simulink model "DZ_DSMC"  (R2021b)
settings: Solver=FixedStepAuto  StartTime=0.0  StopTime=30  FixedStep=1e-5  MaxStep=0.015  RelTol=1e-3
PreLoadFcn:
  | if ~exist('sim_HIL')
  |     sim_HIL=false;
  | end
  | if ~exist('usefilter')
  |     usefilter=false;
  | end
InitFcn:
  | load motorModel.mat
  | load expsetup
model workspace (MAT data in the model file):
  C = Simulink.Parameter
  C.Value = Simulink.data.Expression
  C.Value.ExpressionString = "single(Cs(nodeID,:))"
  C.DataType = 'single'
  C.Complexity = 'real'
  C.Dimensions = -1
  Gam = Simulink.Parameter
  Gam.Value = Simulink.data.Expression
  Gam.Value.ExpressionString = "single(mModel{nodeID,3}.B)"
  Gam.DataType = 'single'
  Gam.Complexity = 'real'
  Gam.Dimensions = -1
  Phi = Simulink.Parameter
  Phi.Value = Simulink.data.Expression
  Phi.Value.ExpressionString = "single(mModel{nodeID,3}.A)"
  Phi.DataType = 'single'
  Phi.Complexity = 'real'
  Phi.Dimensions = -1
  del = Simulink.Parameter
  del.Value = Simulink.data.Expression
  del.Value.ExpressionString = "single(dels(nodeID))"
  del.DataType = 'single'
  del.Complexity = 'real'
  del.Dimensions = -1
  eta = Simulink.Parameter
  eta.Value = Simulink.data.Expression
  eta.Value.ExpressionString = "single(etas(nodeID))"
  eta.DataType = 'single'
  eta.Complexity = 'real'
  eta.Dimensions = -1
  gamm = Simulink.Parameter
  gamm.Value = Simulink.data.Expression
  gamm.Value.ExpressionString = "round(gamms(nodeID))"
  gamm.DataType = 'single'
  gamm.Complexity = 'real'
  gamm.Dimensions = -1
  qT = Simulink.Parameter
  qT.Value = Simulink.data.Expression
  qT.Value.ExpressionString = "single(qTs(nodeID))"
  qT.DataType = 'single'
  qT.Complexity = 'real'
  qT.Dimensions = -1
  vphi = Simulink.Parameter
  vphi.Value = Simulink.data.Expression
  vphi.Value.ExpressionString = "single(vphis(nodeID))"
  vphi.DataType = 'single'
  vphi.Complexity = 'real'
  vphi.Dimensions = -1
  xiT = Simulink.Parameter
  xiT.Value = Simulink.data.Expression
  xiT.Value.ExpressionString = "single(xiTs(nodeID))"
  xiT.DataType = 'single'
  xiT.Complexity = 'real'
  xiT.Dimensions = -1
undefined symbols (not defined in the file): DiscIntNeverNeededParam, N, nodeID, ss_sys, Ts, x607325_PPR
libraries: simulink x1
settings Model: DataDictionary=MotorInfo.sldd  SimulationMode=accelerator  CodeVerificationMode=processor-in-the-loop (pil)  ExtModeTrigDuration=2  Creator=khoi  LastModifiedBy=khoi
settings SolverCC: AlgebraicLoopSolver=TrustRegion  AutoInsertRateTranBlk=on
settings DataIOCC: ExternalInput=i1, i2  LoadExternalInput=on  SaveOutput=off  SaveTime=off
settings OptimizationCC: UseDivisionForNetSlopeComputation=on  GainParamInheritBuiltInType=on  UseFloatMulNetSlope=on  DefaultUnderspecifiedDataType=single  UseSpecifiedMinMax=on  StrengthReduction=on  BitwiseOrLogicalOp=Bitwise operator  PassReuseOutputArgsAs=Individual arguments  NoFixptDivByZeroProtection=on  EfficientFloat2IntCast=on  LifeSpan=inf  MaxStackSize=1024  OptimizeBlockOrder=speed  DifferentSizesBufferReuse=on  OptimizationPriority=Speed  MultiThreadedLoops=on  EfficientTunableParamExpr=on
settings DebuggingCC: SignalInfNanChecking=error  AlgebraicLoopMsg=none  IntegerOverflowMsg=error  ParameterTunabilityLossMsg=error  AssertControl=DisableAll  SFUndirectedBroadcastEventsDiag=error  SFMachineParentedDataDiag=warning
settings HardwareCC: ProdLongLongMode=on
settings ModelReferenceCC: EnableParallelModelReferenceBuilds=on  PropagateVarSize=During execution
settings SFSimCC: CompileTimeRecursionLimit=0  EnableRuntimeRecursion=off  MATLABDynamicMemAlloc=off
settings RTWCC: Description=Embedded Coder  SystemTargetFile=ert.tlc  TemplateMakefile=ert_default_tmf  Toolchain=MinGW64 | gmake (64-bit Windows)  BuildConfiguration=Faster Runs
settings CodeAppCC: ForceParamTrailComments=on  IgnoreCustomStorageClasses=off  OperatorAnnotations=on  SimulinkDataObjDesc=on  SFDataObjDesc=on  MATLABFcnDesc=on  InsertBlockDesc=on
settings ERTTargetCC: TargetLangStandard=C99 (ISO)  CodeReplacementLibrary=GNU C99 extensions  UtilityFuncGeneration=Shared location  CombineSignalStateStructs=on  CodeInterfacePackaging=Reusable function  SupportNonFinite=off  SupportComplex=off  ParenthesesLevel=Maximum  CastingMode=Standards  GenerateAllocFcn=on  GenerateSharedConstants=off  ExtModeTransport=3  ExtModeStaticAlloc=on  ExtModeStaticAllocSize=2048  ExtModeMexFile=ext_xcp  ExtModeIntrfLevel=Level2 - Open  RootIOFormat=Part of model data structure  ERTCustomFileTemplate=example_file_process.tlc

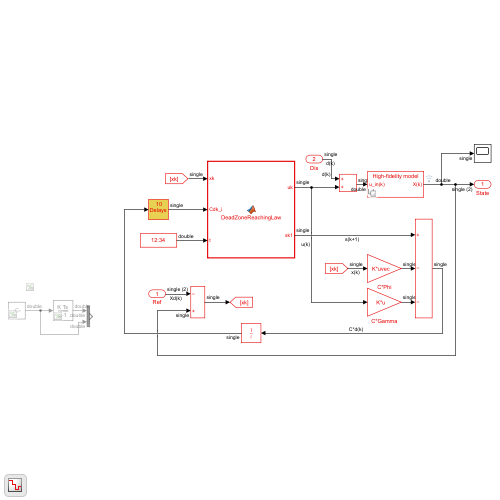
[thumbnail: Simulink's stored preview of the top-level diagram]
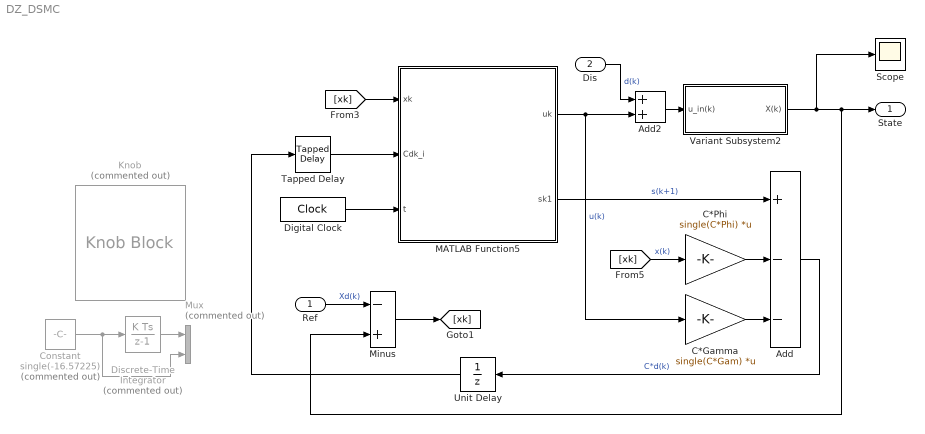
== system DZ_DSMC ==
  Ref : Inport  OutDataTypeStr=single  PortDimensions=2
  Dis : Inport  Port=2  OutDataTypeStr=single  PortDimensions=1
  Add : Sum  Inputs=+--
  Add2 : Sum  OutDataTypeStr=single
  C*Gamma : Gain  Gain=single(C*Gam)  Multiplication=Matrix(K*u)
  C*Phi : Gain  Gain=single(C*Phi)  Multiplication=Matrix(K*u) (u vector)
  Constant : Constant  Commented=on  Value=single(-16.57225)  SampleTime=Ts
  Digital Clock : DigitalClock  SampleTime=Ts
  Discrete-Time Integrator : DiscreteIntegrator  Commented=on  SampleTime=-1  ICPrevOutput=DiscIntNeverNeededParam  ICPrevScaledInput=DiscIntNeverNeededParam
  Knob : KnobBlock  Commented=on  ScaleMin=-50  ScaleMax=50
  MATLAB Function5 : MATLAB Function  TreatAsAtomicUnit=on  mask{Phi=single(Phi), Gam=single(Gam), C=single(C), qT=single(qT), xiT=single(xiT), del=single(del), vphi=single(vphi), gamm=uint8(gamm), eta=single(eta), Ts=single(Ts), n=uint8(N)}
      mask prompts: Gam "Gamma"; C "Sliding vector"; qT "qT (0<1-qT<1)"; xiT "xiT>0"; del "0<delta<1"; vphi "vphi>0"; gamm "gamma (natural num +)"; eta "eta>0"
  Minus : Sum  Inputs=-+
  Mux : Mux  Commented=on  Inputs=2
  Scope : Scope
  Tapped Delay : simulink/Discrete/Tapped Delay  vinit=0.0  samptime=-1  NumDelays=N  DelayOrder=Newest  includeCurrent=on
  Unit Delay : UnitDelay  SampleTime=-1  HasFrameUpgradeWarning=on
  Variant Subsystem2 : Subsystem  Variant=on  mask{Phi=single(Phi), Gam=single(Gam), NodeID=nodeID, Ts=single(Ts)}
      mask prompts: Phi "State matrix"; Gam "Input matrix"; NodeID "node ID"; Ts "Sample time (s)"
      mask init:
      | myDictionaryObj = Simulink.data.dictionary.open('MotorInfo.sldd');
      mask DialogControl ParameterGroupVar Prompt: Mathematical model
      mask DialogControl ParameterGroupVar_copy Prompt: Mathematical model
  State : Outport  OutDataTypeStr=single  PortDimensions=2
  wires:
  Minus/1 -> [xk]
  Add/1 -> Unit Delay/1  "C*d(k)"
  MATLAB Function5/1(uk) -> C*Gamma/1, Add2/2  "u(k)"
  [xk] -> MATLAB Function5/1(xk)
  [xk] -> C*Phi/1  "x(k)"
  MATLAB Function5/2(sk1) -> Add/1  "s(k+1)"
  C*Gamma/1 -> Add/3
  C*Phi/1 -> Add/2
  Tapped Delay/1 -> MATLAB Function5/2(Cdk_i)
  Dis/1 -> Add2/1  "d(k)"
  Unit Delay/1 -> Tapped Delay/1
  Digital Clock/1 -> MATLAB Function5/3(t)
  Ref/1 -> Minus/1  "Xd(k)"
  Discrete-Time Integrator/1 -> Mux/1
  Constant/1 -> Mux/2, Discrete-Time Integrator/1
  Variant Subsystem2/1(X(k)) -> Scope/1, Minus/2, State/1
  Add2/1 -> Variant Subsystem2/1(u_in(k))

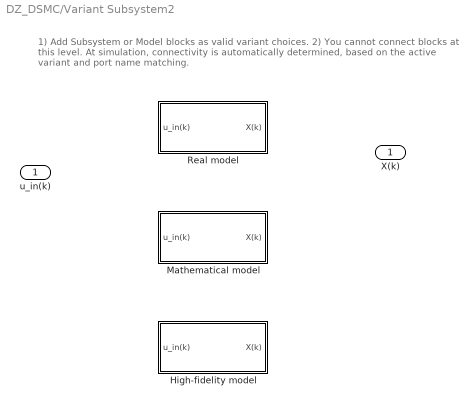
== system DZ_DSMC/Variant Subsystem2 ==
  note: 1) Add Subsystem or Model blocks as valid variant choices.
      | 2) You cannot connect blocks at this level. At simulation, connectivity is automatically
      | determined, based on the active variant and port name matching.
  u_in(k) : Inport
  High-fidelity model : Subsystem  VariantControl=simMode == 1
  Mathematical model : Subsystem  VariantControl=simMode == 0
  Real model : Subsystem  VariantControl=simMode == 2
  X(k) : Outport

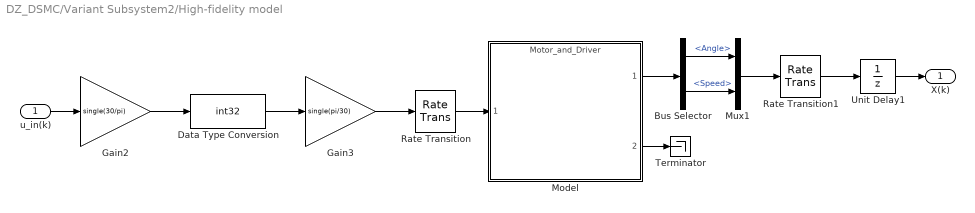
== system DZ_DSMC/Variant Subsystem2/High-fidelity model ==
  u_in(k) : Inport
  Bus Selector : BusSelector  OutputSignals=Angle,Speed
  Data Type Conversion : DataTypeConversion  OutDataTypeStr=int32  RndMeth=Simplest
  Gain2 : Gain  Gain=single(30/pi)  ParamDataTypeStr=Inherit: Same as input
  Gain3 : Gain  Gain=single(pi/30)  ParamDataTypeStr=single
  Model : ModelReference  ModelNameDialog=Motor_and_Driver.slx  ModelReferenceVersion=4.61
  Mux1 : Mux  Inputs=2
  Rate Transition : RateTransition
  Rate Transition1 : RateTransition
  Terminator : Terminator
  Unit Delay1 : UnitDelay  SampleTime=-1  HasFrameUpgradeWarning=on
  X(k) : Outport  OutDataTypeStr=single
  wires:
  Model/2 -> Terminator/1
  u_in(k)/1 -> Gain2/1
  Data Type Conversion/1 -> Gain3/1
  Gain2/1 -> Data Type Conversion/1
  Rate Transition/1 -> Model/1
  Model/1 -> Bus Selector/1
  Mux1/1 -> Rate Transition1/1
  Gain3/1 -> Rate Transition/1
  Bus Selector/1 -> Mux1/1  "<Angle>"
  Bus Selector/2 -> Mux1/2  "<Speed>"
  Rate Transition1/1 -> Unit Delay1/1
  Unit Delay1/1 -> X(k)/1

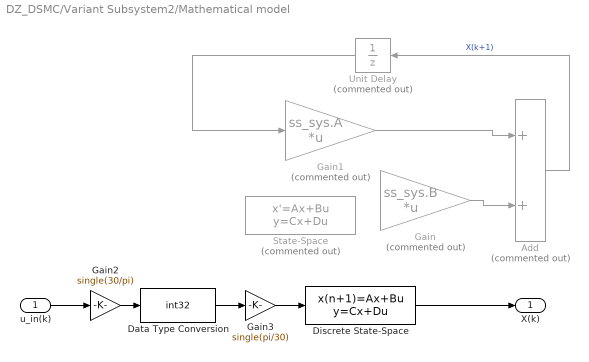
== system DZ_DSMC/Variant Subsystem2/Mathematical model ==
  u_in(k) : Inport
  Add : Sum  Commented=on
  Data Type Conversion : DataTypeConversion  OutDataTypeStr=int32  RndMeth=Simplest
  Discrete State-Space : DiscreteStateSpace  A=Phi  B=Gam  C=[1 0; 0 1]  D=zeros(2,1)  SampleTime=-1
  Gain : Gain  Commented=on  Gain=ss_sys.B  Multiplication=Matrix(K*u) (u vector)
  Gain1 : Gain  Commented=on  Gain=ss_sys.A  Multiplication=Matrix(K*u) (u vector)
  Gain2 : Gain  Gain=single(30/pi)  ParamDataTypeStr=Inherit: Same as input
  Gain3 : Gain  Gain=single(pi/30)  ParamDataTypeStr=single
  State-Space : StateSpace  Commented=on  A=ss_sys.A  B=ss_sys.B  C=eye(2)  D=[0;0]  InitialCondition=0
  Unit Delay : UnitDelay  Commented=on  SampleTime=-1  HasFrameUpgradeWarning=on
  X(k) : Outport  OutDataTypeStr=single
  wires:
  Add/1 -> Unit Delay/1  "X(k+1)"
  Gain1/1 -> Add/1
  Unit Delay/1 -> Gain1/1
  Gain/1 -> Add/2
  u_in(k)/1 -> Gain2/1
  Discrete State-Space/1 -> X(k)/1
  Gain2/1 -> Data Type Conversion/1
  Gain3/1 -> Discrete State-Space/1
  Data Type Conversion/1 -> Gain3/1

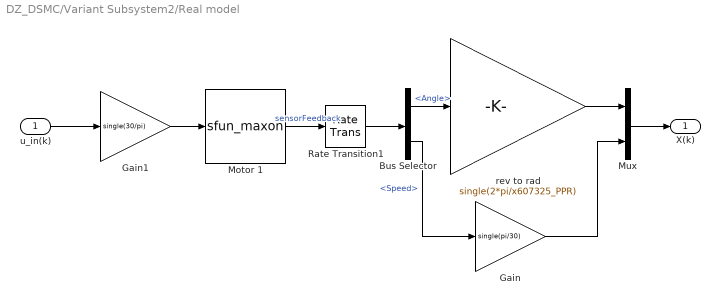
== system DZ_DSMC/Variant Subsystem2/Real model ==
  u_in(k) : Inport  OutDataTypeStr=single
  Bus Selector : BusSelector  OutputSignals=Angle,Speed
  Gain : Gain  Gain=single(pi/30)
  Gain1 : Gain  Gain=single(30/pi)  RndMeth=Simplest
  Motor 1 : S-Function  FunctionName=sfun_maxon  Parameters=NodeID, DeltaT, OpMode  SFunctionDeploymentMode=off  EnableBusSupport=off  mask{NodeID=NodeID, DeltaT=double(0.015), OpMode=Cyclic synchronous velocity mode, P_cur=0, I_cur=0, P_pos=0, I_pos=0, D_pos=0, v_posGainFF=0, a_posGainFF=0, P_vel=0, I_vel=0, v_velGainFF=0, a_velGainFF=0, f_velCutoff=0}
      mask prompts: NodeID "Node ID"; DeltaT "Sample time (s)"; OpMode "Operation mode"; P_cur "P gain"; I_cur "I gain"; P_pos "P gain"; I_pos "I gain"; D_pos "D gain"; v_posGainFF "FF velocity gain"; a_posGainFF "FF acceleration gain"; P_vel "P gain"; I_vel "I gain"; v_velGainFF "Feed-forward velocity gain"; a_velGainFF "Feed-forward acceleration gain"; f_velCutoff "Filter cut-off frequency"
      mask TypeOptions OpMode: Cyclic synchronous current (torque) mode | Cyclic synchronous velocity mode | Cyclic synchronous position mode | Profile velocity mode | Profile position mode
      mask DialogControl DescGroupVar Prompt: Motor Parameters
      mask DialogControl DescTextVar Prompt: The block outputs MotorInfo bus signal, which consists of the following variables: angle (increment), speed (rpm), current (mA)
      mask DialogControl Container6 Prompt: Motor
      mask DialogControl Container14 Prompt: Controller Parameters
      mask DialogControl DescTextVar_copy Prompt: This tab is experimental and does not implemented yet. Changing these parameters will not affect the motor performance.
      mask DialogControl Container15 Prompt: Current controller parameter set
      mask DialogControl Container15_copy Prompt: Position controller parameter set
      mask DialogControl Container15_copy_copy Prompt: Velocity controller parameter set
      mask Display:
      | disp('Maxon motor\nHIL');
      | % port_label('input', 1, 'inputSignal');
      | % port_label('output', 1, 'SENSR');
  Mux : Mux  Inputs=2
  Rate Transition1 : RateTransition
  rev to rad : Gain  Gain=single(2*pi/x607325_PPR)
  X(k) : Outport  OutDataTypeStr=single
  wires:
  u_in(k)/1 -> Gain1/1
  rev to rad/1 -> Mux/1
  Bus Selector/2 -> Gain/1  "<Speed>"
  Gain1/1 -> Motor 1/1
  Motor 1/1 -> Rate Transition1/1  "sensorFeedback"
  Rate Transition1/1 -> Bus Selector/1
  Gain/1 -> Mux/2
  Bus Selector/1 -> rev to rad/1  "<Angle>"
  Mux/1 -> X(k)/1

== matlab function DZ_DSMC/MATLAB Function5 ==
  data: xk input; uk output single; Cdk_i input; t input; Phi parameter single; C parameter single; qT parameter single; xiT parameter single; del parameter single; eta parameter single; gamm parameter single; vphi parameter single; sk1 output single; n parameter single; Ts parameter single; Gam parameter single
function [uk,sk1] = DeadZoneReachingLaw(xk,Cdk_i,t,...
    Phi, C, qT, xiT, del, eta, gamm, vphi, n, Ts, Gam)

% calcualte switching function
sk = C*xk;

% calculate finite number function
persistent k;
if isempty(k)
    k=0;
end
if k<n
    if uint8(ceil(rem(t,Ts)))==0 && uint8(ceil(t))~=0
        k = k+1;
    end
end
vthe = k;

% calculate ud(k) - high-order compensator
udk = single(0);
for i=1:vthe
    udk = udk - (-1)^i*nchoosek(vthe,i)*Cdk_i(i+1);
end

% calculate Lambda(k) - exponential function
Lamk= single(del + (1-del)*exp(-vphi*abs(sk)^gamm));

% calculate rho[s(k)] - dead zone function
if sk>eta
        rhosk=1;
    elseif abs(sk)<=eta
        rhosk=0;
    else % sk<-eta
        rhosk=-1;
end

% calcualte high-order difference function
hodf = Cdk_i(1) - udk;

% calculate one-step forward switching function
sk1 = (1-qT)*Lamk*sk - xiT/Lamk*rhosk + hodf;

% calculate dead zone reaching law controller
uk = -(C*Gam)\(C*Phi*xk - (1-qT)*Lamk*sk + xiT/Lamk*rhosk + udk);
